simulink model "tran_opoz"  (R2016b)
settings: Solver=ode45  StartTime=0.0  StopTime=Tsym  RelTol=1e-3  EnableMultiTasking=on
undefined symbols (not defined in the file): deltaFc, deltaFd, deltaFh, deltaTc, deltaTd, deltaTh, G1, h0, T0, Tciagly, Tskok
settings Model: Creator=Arek  LastModifiedBy=Luke
settings DataIOCC: LimitDataPoints=on  SaveFormat=Array
settings OptimizationCC: LifeSpan=inf
settings DebuggingCC: SFUnexpectedBacktrackingDiag=warning  SFNoUnconditionalDefaultTransitionDiag=warning  SFExecutionAtInitializationDiag=none
settings HardwareCC: ProdBitPerPointer=32  ProdBitPerSizeT=32  ProdBitPerPtrDiffT=32  ProdLargestAtomicFloat=None  ProdIntDivRoundTo=Undefined  ProdEndianess=Unspecified  ProdWordSize=32  ProdHWDeviceType=32-bit Generic
settings ModelReferenceCC: PropagateSignalLabelsOutOfModel=off
settings GRTTargetCC: TargetLangStandard=C89/C90 (ANSI)  GeneratePreprocessorConditionals=Disable all
settings ConfigComp: CovMetricSettings=dw  CovHtmlReporting=on  CovSaveCumulativeToWorkspaceVar=on  CovSaveSingleToWorkspaceVar=on  CovExternalEMLEnable=off  CovSFcnEnable=off

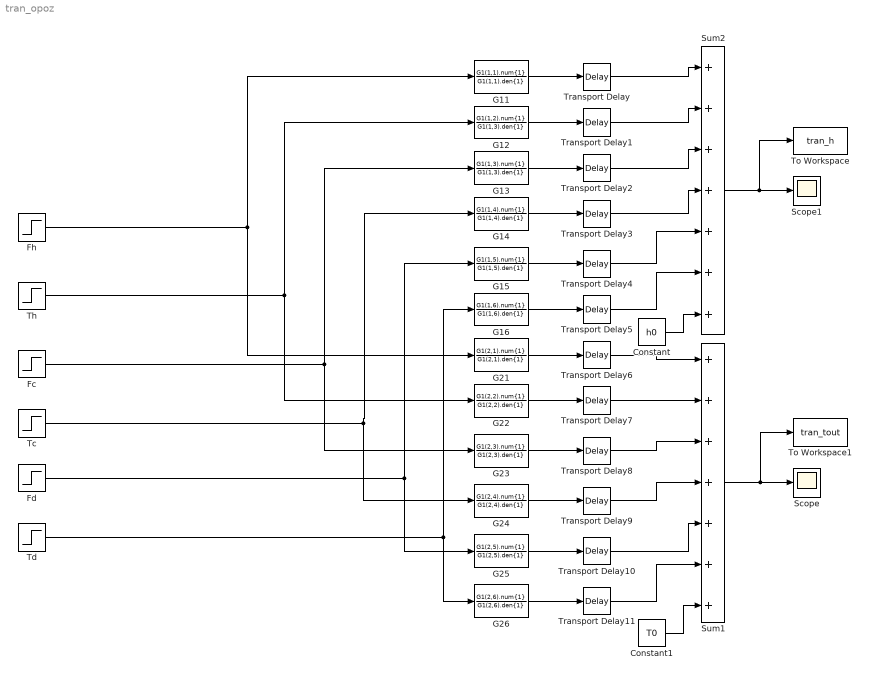
== system tran_opoz ==
  Constant : Constant  Value=h0
  Constant1 : Constant  Value=T0
  Fc : Step  Time=0  After=deltaFc  SampleTime=Tciagly
  Fd : Step  Time=Tskok  After=deltaFd  SampleTime=Tciagly
  Fh : Step  Time=Tskok  After=deltaFh  SampleTime=Tciagly
  G11 : TransferFcn  Numerator=G1(1,1).num{1}  Denominator=G1(1,1).den{1}
  G12 : TransferFcn  Numerator=G1(1,2).num{1}  Denominator=G1(1,3).den{1}
  G13 : TransferFcn  Numerator=G1(1,3).num{1}  Denominator=G1(1,3).den{1}
  G14 : TransferFcn  Numerator=G1(1,4).num{1}  Denominator=G1(1,4).den{1}
  G15 : TransferFcn  Numerator=G1(1,5).num{1}  Denominator=G1(1,5).den{1}
  G16 : TransferFcn  Numerator=G1(1,6).num{1}  Denominator=G1(1,6).den{1}
  G21 : TransferFcn  Numerator=G1(2,1).num{1}  Denominator=G1(2,1).den{1}
  G22 : TransferFcn  Numerator=G1(2,2).num{1}  Denominator=G1(2,2).den{1}
  G23 : TransferFcn  Numerator=G1(2,3).num{1}  Denominator=G1(2,3).den{1}
  G24 : TransferFcn  Numerator=G1(2,4).num{1}  Denominator=G1(2,4).den{1}
  G25 : TransferFcn  Numerator=G1(2,5).num{1}  Denominator=G1(2,5).den{1}
  G26 : TransferFcn  Numerator=G1(2,6).num{1}  Denominator=G1(2,6).den{1}
  Scope : Scope
  Scope1 : Scope
  Sum1 : Sum  Inputs=+++++++
  Sum2 : Sum  Inputs=+++++++
  Tc : Step  Time=Tskok  After=deltaTc  SampleTime=Tciagly
  Td : Step  Time=Tskok  After=deltaTd  SampleTime=Tciagly
  Th : Step  Time=Tskok  After=deltaTh  SampleTime=Tciagly
  To Workspace : ToWorkspace  VariableName=tran_h  SaveFormat=Timeseries  SampleTime=-1
  To Workspace1 : ToWorkspace  VariableName=tran_tout  SaveFormat=Timeseries  SampleTime=-1
  Transport Delay : TransportDelay  DelayTime=G1(1,1).ioDelay
  Transport Delay1 : TransportDelay  DelayTime=G1(1,2).ioDelay
  Transport Delay10 : TransportDelay  DelayTime=G1(2,5).ioDelay
  Transport Delay11 : TransportDelay  DelayTime=G1(2,6).ioDelay
  Transport Delay2 : TransportDelay  DelayTime=G1(1,3).ioDelay
  Transport Delay3 : TransportDelay  DelayTime=G1(1,4).ioDelay
  Transport Delay4 : TransportDelay  DelayTime=G1(1,5).ioDelay
  Transport Delay5 : TransportDelay  DelayTime=G1(1,6).ioDelay
  Transport Delay6 : TransportDelay  DelayTime=G1(2,1).ioDelay
  Transport Delay7 : TransportDelay  DelayTime=G1(2,2).ioDelay
  Transport Delay8 : TransportDelay  DelayTime=G1(2,3).ioDelay
  Transport Delay9 : TransportDelay  DelayTime=G1(2,4).ioDelay
  wires:
  Fh/1 -> G11/1, G21/1
  Th/1 -> G12/1, G22/1
  Fc/1 -> G13/1, G23/1
  Tc/1 -> G14/1, G24/1
  Fd/1 -> G25/1, G15/1
  Td/1 -> G26/1, G16/1
  G23/1 -> Transport Delay8/1
  G11/1 -> Transport Delay/1
  G12/1 -> Transport Delay1/1
  G13/1 -> Transport Delay2/1
  G14/1 -> Transport Delay3/1
  G15/1 -> Transport Delay4/1
  G16/1 -> Transport Delay5/1
  G21/1 -> Transport Delay6/1
  G22/1 -> Transport Delay7/1
  G24/1 -> Transport Delay9/1
  G25/1 -> Transport Delay10/1
  G26/1 -> Transport Delay11/1
  Transport Delay6/1 -> Sum1/1
  Transport Delay7/1 -> Sum1/2
  Transport Delay5/1 -> Sum2/6
  Transport Delay4/1 -> Sum2/5
  Transport Delay3/1 -> Sum2/4
  Transport Delay2/1 -> Sum2/3
  Transport Delay1/1 -> Sum2/2
  Transport Delay/1 -> Sum2/1
  Transport Delay11/1 -> Sum1/6
  Transport Delay10/1 -> Sum1/5
  Transport Delay9/1 -> Sum1/4
  Transport Delay8/1 -> Sum1/3
  Sum1/1 -> To Workspace1/1, Scope/1
  Sum2/1 -> To Workspace/1, Scope1/1
  Constant/1 -> Sum2/7
  Constant1/1 -> Sum1/7
